simulink model "skateboard_model"  (R2017b)
settings: Solver=VariableStepAuto  StartTime=0.0  StopTime=30  RelTol=1e-3
undefined symbols (not defined in the file or in its folder): cycle, magnitude, vehicle
settings Model: Creator=bahlmann  LastModifiedBy=bahlmann

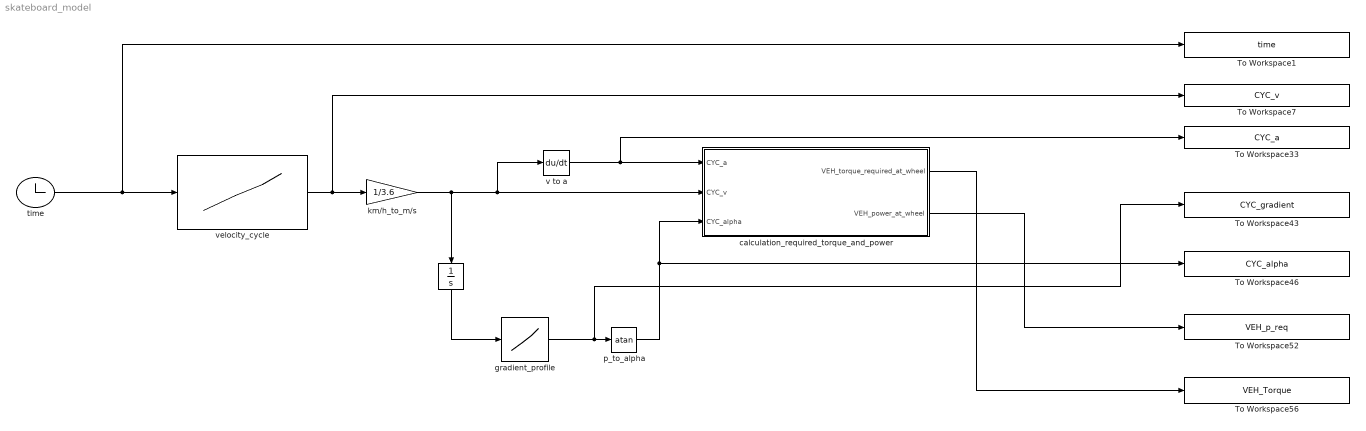
== system skateboard_model ==
  "    " : Integrator
  To Workspace1 : ToWorkspace  VariableName=time  SampleTime=-1
  To Workspace33 : ToWorkspace  VariableName=CYC_a  SampleTime=-1
  To Workspace43 : ToWorkspace  VariableName=CYC_gradient  SampleTime=-1
  To Workspace46 : ToWorkspace  VariableName=CYC_alpha  SampleTime=-1
  To Workspace52 : ToWorkspace  VariableName=VEH_p_req  SampleTime=-1
  To Workspace56 : ToWorkspace  VariableName=VEH_Torque  SampleTime=-1
  To Workspace7 : ToWorkspace  VariableName=CYC_v  SampleTime=-1
  calculation_required_torque_and_power : Subsystem
  gradient_profile : Lookup  InputValues=cycle.gradient_vs_distance(:,1)  Table=cycle.gradient_vs_distance(:,2)  SaturateOnIntegerOverflow=on
  km/h_to_m/s : Gain  Gain=1/3.6
  p_to_alpha : Trigonometry  Operator=atan
  time : Clock
  "v to a " : Derivative
  velocity_cycle : Lookup_n-D  RequirementInfo={} %GIDa_a1a33fa5_7431_45ee_992e_6b114a650843  NumberOfTableDimensions=1  BreakpointsForDimension1=cycle.speed(:,1)  Table=cycle.speed(:,2)  RndMeth=Simplest  InputSameDT=on
  wires:
  time/1 -> To Workspace1/1, velocity_cycle/1
  velocity_cycle/1 -> To Workspace7/1, km/h_to_m/s/1
  km/h_to_m/s/1 -> "v to a "/1, calculation_required_torque_and_power/2(CYC_v), "    "/1
  "v to a "/1 -> To Workspace33/1, calculation_required_torque_and_power/1(CYC_a)
  "    "/1 -> gradient_profile/1
  gradient_profile/1 -> To Workspace43/1, p_to_alpha/1
  p_to_alpha/1 -> To Workspace46/1, calculation_required_torque_and_power/3(CYC_alpha)
  calculation_required_torque_and_power/2(VEH_power_at_wheel) -> To Workspace52/1
  calculation_required_torque_and_power/1(VEH_torque_required_at_wheel) -> To Workspace56/1

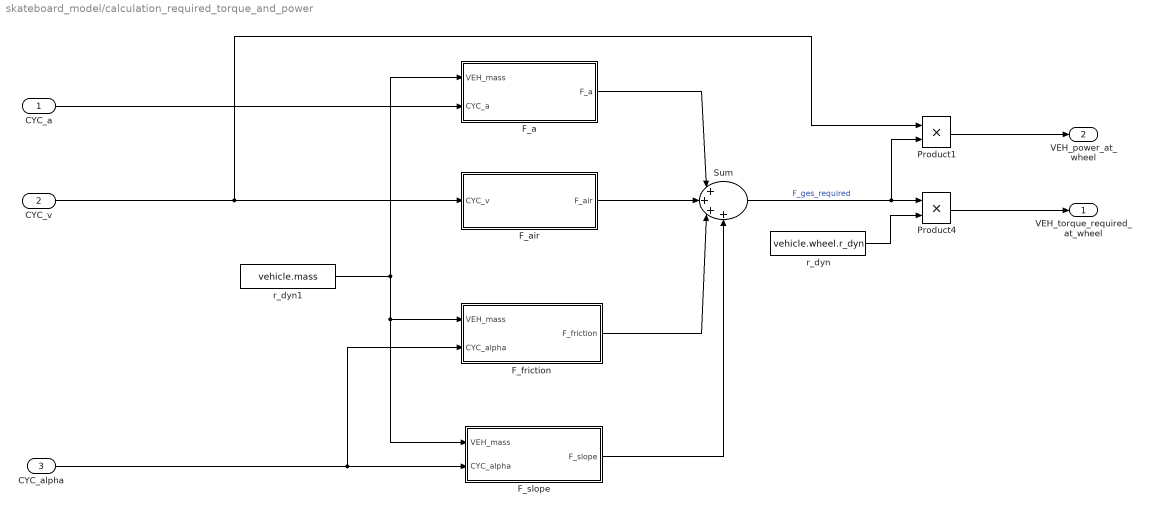
== system skateboard_model/calculation_required_torque_and_power ==
  CYC_a : Inport
  CYC_v : Inport  Port=2
  CYC_alpha : Inport  Port=3
  F_a : Subsystem
  F_air : Subsystem
  F_friction : Subsystem
  "F_slope " : Subsystem
  Product1 : Product  RndMeth=Zero
  Product4 : Product  RndMeth=Zero
  Sum : Sum  Inputs=|++++
  r_dyn : Constant  Value=vehicle.wheel.r_dyn
  r_dyn1 : Constant  Value=vehicle.mass
  VEH_torque_required_at_wheel : Outport
  VEH_power_at_wheel : Outport  Port=2
  wires:
  r_dyn1/1 -> "F_slope "/1(VEH_mass), F_friction/1(VEH_mass), F_a/1(VEH_mass)
  F_a/1(F_a) -> Sum/1
  CYC_a/1 -> F_a/2(CYC_a)
  F_air/1(F_air) -> Sum/2
  CYC_v/1 -> Product1/1, F_air/1(CYC_v)
  F_friction/1(F_friction) -> Sum/3
  "F_slope "/1(F_slope) -> Sum/4
  CYC_alpha/1 -> F_friction/2(CYC_alpha), "F_slope "/2(CYC_alpha)
  Product4/1 -> VEH_torque_required_at_wheel/1
  r_dyn/1 -> Product4/2
  Sum/1 -> Product1/2, Product4/1  "F_ges_required"
  Product1/1 -> VEH_power_at_wheel/1

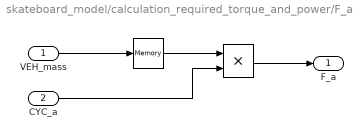
== system skateboard_model/calculation_required_torque_and_power/F_a ==
  VEH_mass : Inport
  CYC_a : Inport  Port=2
  " " : Memory
  "  " : Product  RndMeth=Zero
  F_a : Outport
  wires:
  CYC_a/1 -> "  "/2
  " "/1 -> "  "/1
  "  "/1 -> F_a/1
  VEH_mass/1 -> " "/1

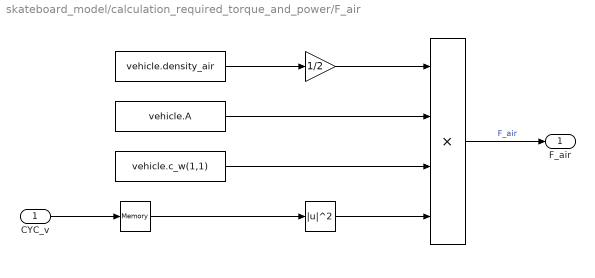
== system skateboard_model/calculation_required_torque_and_power/F_air ==
  CYC_v : Inport
  " " : Gain  Gain=1/2
  "  " : Memory
  "   " : Math  Operator=magnitude^2  SaturateOnIntegerOverflow=on
  "    " : Product  Inputs=4  RndMeth=Zero
  " " : Constant  Value=vehicle.density_air
  " " : Constant  Value=vehicle.A
  " " : Constant  Value=vehicle.c_w(1,1)
  F_air : Outport
  wires:
  "  "/1 -> "   "/1
  "    "/1 -> F_air/1  "F_air"
  CYC_v/1 -> "  "/1
  "   "/1 -> "    "/4
  " "/1 -> "    "/3
  " "/1 -> "    "/2
  " "/1 -> "    "/1
  " "/1 -> " "/1

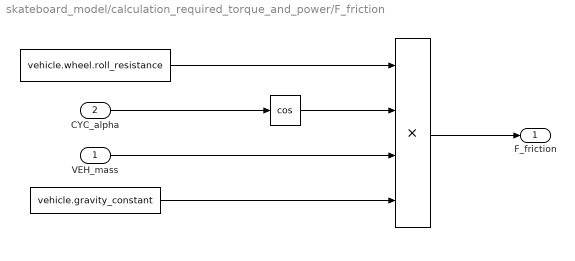
== system skateboard_model/calculation_required_torque_and_power/F_friction ==
  VEH_mass : Inport
  CYC_alpha : Inport  Port=2
  " " : Trigonometry  Operator=cos
  "  " : Constant  Value=vehicle.gravity_constant
  "   " : Product  Inputs=4  RndMeth=Zero
  " " : Constant  Value=vehicle.wheel.roll_resistance
  F_friction : Outport
  wires:
  CYC_alpha/1 -> " "/1
  " "/1 -> "   "/2
  VEH_mass/1 -> "   "/3
  "  "/1 -> "   "/4
  "   "/1 -> F_friction/1
  " "/1 -> "   "/1

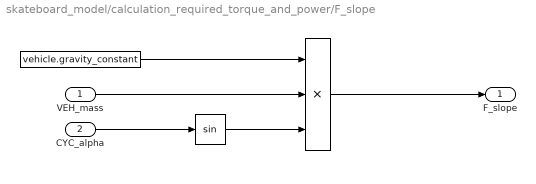
== system skateboard_model/calculation_required_torque_and_power/F_slope  ==
  VEH_mass : Inport
  CYC_alpha : Inport  Port=2
  " " : Trigonometry
  "  " : Constant  Value=vehicle.gravity_constant
  "    " : Product  Inputs=3  RndMeth=Zero
  F_slope : Outport
  wires:
  CYC_alpha/1 -> " "/1
  VEH_mass/1 -> "    "/2
  "  "/1 -> "    "/1
  " "/1 -> "    "/3
  "    "/1 -> F_slope/1
